simulink model "B"  (R2021a)
settings: Solver=VariableStepAuto  StartTime=0.0  StopTime=10.0  RelTol=1e-3
values from neighbouring files (symbols this model uses):
  C1 = 1    [untitled.m]
  C2 = 1    [untitled.m]
  R1 = 1    [untitled.m]
  R2 = 1    [untitled.m]
  x = 1    [untitled.m]
libraries: simulink x2, simulink_extras x2
settings Model: Creator=solo  LastModifiedBy=solo

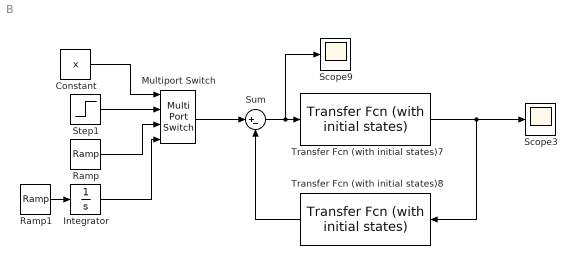
== system B ==
  Constant : Constant  Value=x
  Integrator : Integrator
  Multiport Switch : MultiPortSwitch
  Ramp : simulink/Sources/Ramp  slope=1  start=0  InitialOutput=0
  Ramp1 : simulink/Sources/Ramp  slope=1  start=0  InitialOutput=0
  Scope3 : Scope
  Scope9 : Scope
  Step1 : Step  Time=0  SampleTime=0
  Sum : Sum  Inputs=|+-
  Transfer Fcn (with initial states)7 : simulink_extras/Additional Linear/Transfer Fcn (with initial states)  N="[ (C2*R2)    1]"  D="[ (R1*R2*C1*C2 )    (R1*C2+R1*C1)      0]"  X0=0
  Transfer Fcn (with initial states)8 : simulink_extras/Additional Linear/Transfer Fcn (with initial states)  N=[1]  D=[1]  X0=0
  wires:
  Constant/1 -> Multiport Switch/1
  Sum/1 -> Scope9/1, Transfer Fcn (with initial states)7/1
  Multiport Switch/1 -> Sum/1
  Ramp1/1 -> Integrator/1
  Ramp/1 -> Multiport Switch/3
  Integrator/1 -> Multiport Switch/4
  Step1/1 -> Multiport Switch/2
  Transfer Fcn (with initial states)7/1 -> Transfer Fcn (with initial states)8/1, Scope3/1
  Transfer Fcn (with initial states)8/1 -> Sum/2
